simulink model "sim"  (R2022b)
settings: Solver=FixedStepAuto  StartTime=0.0  StopTime=20  FixedStep=0.01  RelTol=1e-3
values from neighbouring files (symbols this model uses):
  A = double(vpa(subs(A, [x, Parameter, u], [xe, Parameter_value, 0]), 10))    [lqr_cartpole.m]
  B = double(vpa(subs(B, [x, Parameter, u], [xe, Parameter_value, 0]), 10))    [lqr_cartpole.m]
  C = double(C)    [lqr_cartpole.m]
  KD = 0.015    [lqr_cartpole.m]
  KP = 0.15    [lqr_cartpole.m]
  L1 = place(A.',C.',poles_ob).'    [lqr_cartpole.m]
undefined symbols (not defined in the file or in its folder): K_LQR
settings Model: Creator=mehti  LastModifiedBy=MMM
settings SolverCC: AlgebraicLoopSolver=TrustRegion
settings DebuggingCC: UnconnectedInputMsg=warning  UnconnectedOutputMsg=warning  UnconnectedLineMsg=warning  SFMachineParentedDataDiag=warning
settings ModelReferenceCC: EnableRefExpFcnMdlSchedulingChecks=on
settings RTWCC: DLArmComputeVersion=19.05

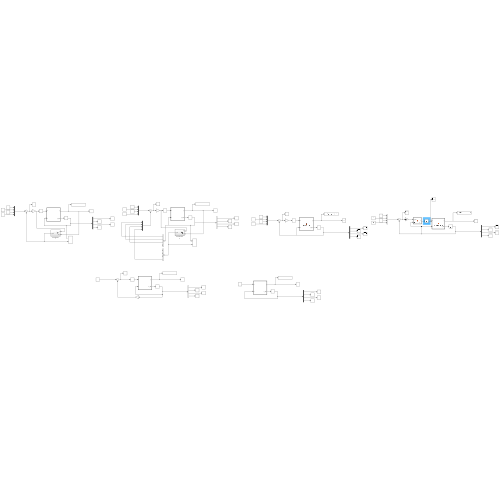
[thumbnail: Simulink's stored preview of the top-level diagram]
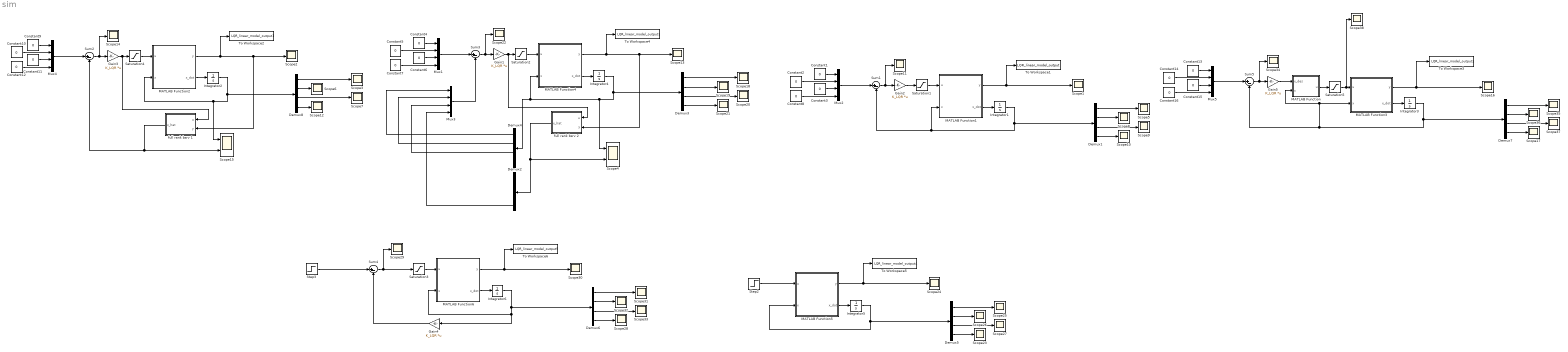
== system sim ==
  Constant{1..16} (16 alike) : Constant  Value=0
  Demux{1..8} (8 alike) : Demux
  Gain{1..5} (5 alike) : Gain  Gain=K_LQR  Multiplication=Matrix(K*u)
  Integrator{1..6} (6 alike) : Integrator  InitialCondition=[0, 0, pi/8 ,0]
  MATLAB Function : MATLAB Function  TreatAsAtomicUnit=on
  MATLAB Function1 : MATLAB Function  TreatAsAtomicUnit=on
  MATLAB Function2 : MATLAB Function  TreatAsAtomicUnit=on
  MATLAB Function3 : MATLAB Function  TreatAsAtomicUnit=on
  MATLAB Function4 : MATLAB Function  TreatAsAtomicUnit=on
  MATLAB Function5 : MATLAB Function  TreatAsAtomicUnit=on
  MATLAB Function6 : MATLAB Function  TreatAsAtomicUnit=on
  Mux{1..5} (5 alike) : Mux
  Saturation{1..4} (4 alike) : Saturate  UpperLimit=10  LowerLimit=-10
  Saturation5 : Saturate  UpperLimit=1000  LowerLimit=-1000
  Scope{1..3,5..14,16..38} (36 alike) : Scope
  Scope15 : Scope  NumInputPorts=2
  Scope4 : Scope  NumInputPorts=2
  Step2 : Step  Time=0.5  After=0  SampleTime=0
  Step3 : Step  Time=0.5  After=0.2  SampleTime=0
  Sum{1..5} (5 alike) : Sum  Inputs=|+-
  To Workspace1 : ToWorkspace  VariableName=LQR_linear_model_output  SaveFormat=Timeseries  SampleTime=-1
  To Workspace2 : ToWorkspace  VariableName=LQR_linear_model_output1  SaveFormat=Timeseries  SampleTime=-1
  To Workspace3 : ToWorkspace  VariableName=LQR_linear_model_output2  SaveFormat=Timeseries  SampleTime=-1
  To Workspace4 : ToWorkspace  VariableName=LQR_linear_model_output3  SaveFormat=Timeseries  SampleTime=-1
  To Workspace5 : ToWorkspace  VariableName=LQR_linear_model_output4  SaveFormat=Timeseries  SampleTime=-1
  To Workspace6 : ToWorkspace  VariableName=LQR_linear_model_output5  SaveFormat=Timeseries  SampleTime=-1
  full rank bsrv 1 : Subsystem
  full rank bsrv 2 : Subsystem
  wires:
  Saturation2/1 -> MATLAB Function4/1(u)
  Constant7/1 -> Mux1/4
  Constant5/1 -> Mux1/2
  Constant6/1 -> Mux1/3
  Constant4/1 -> Mux1/1
  Demux3/1 -> Scope18/1
  Demux3/2 -> Scope19/1
  Demux3/3 -> Scope20/1
  Demux3/4 -> Scope21/1
  Gain1/1 -> full rank bsrv 2/1(u), Saturation2/1
  Integrator4/1 -> Scope4/1, Demux4/1, MATLAB Function4/2(x), Demux3/1
  Sum3/1 -> Gain1/1, Scope22/1
  MATLAB Function4/2(x_dot) -> Integrator4/1
  MATLAB Function4/1(y) -> To Workspace4/1, full rank bsrv 2/2(y), Scope13/1
  Mux1/1 -> Sum3/1
  Step2/1 -> MATLAB Function5/1(u)
  Demux5/1 -> Scope25/1
  Demux5/2 -> Scope26/1
  Demux5/3 -> Scope27/1
  MATLAB Function5/2(x_dot) -> Integrator5/1
  Integrator5/1 -> Demux5/1, MATLAB Function5/2(x)
  Demux5/4 -> Scope23/1
  MATLAB Function5/1(y) -> Scope24/1, To Workspace5/1
  Step3/1 -> Sum4/1
  Gain4/1 -> Sum4/2
  MATLAB Function6/1(y) -> To Workspace6/1, Scope30/1
  Demux6/4 -> Scope28/1
  Integrator6/1 -> MATLAB Function6/2(x), Gain4/1, Demux6/1
  MATLAB Function6/2(x_dot) -> Integrator6/1
  Demux6/3 -> Scope33/1
  Demux6/2 -> Scope32/1
  Saturation3/1 -> MATLAB Function6/1(u)
  Demux6/1 -> Scope31/1
  Sum4/1 -> Scope29/1, Saturation3/1
  full rank bsrv 2/1(x_hat) -> Demux2/1, Scope4/2
  Demux4/1 -> Mux3/1
  Demux4/2 -> Mux3/2
  Demux4/3 -> Mux3/3
  Demux2/4 -> Mux3/4
  Mux3/1 -> Sum3/2
  Constant8/1 -> Mux2/4
  Demux1/2 -> Scope8/1
  Constant2/1 -> Mux2/2
  Saturation1/1 -> MATLAB Function1/1(u)
  Constant3/1 -> Mux2/3
  Constant1/1 -> Mux2/1
  Demux1/3 -> Scope9/1
  Sum1/1 -> Scope11/1, Gain2/1
  Demux1/1 -> Scope5/1
  Integrator1/1 -> Demux1/1, MATLAB Function1/2(x), Sum1/2
  MATLAB Function1/1(y) -> Scope1/1, To Workspace1/1
  Demux1/4 -> Scope10/1
  MATLAB Function1/2(x_dot) -> Integrator1/1
  Gain2/1 -> Saturation1/1
  Mux2/1 -> Sum1/1
  full rank bsrv 1/1(x_hat) -> Sum2/2, Scope15/2
  Mux4/1 -> Sum2/1
  MATLAB Function2/1(y) -> Scope2/1, full rank bsrv 1/2(y), To Workspace2/1
  MATLAB Function2/2(x_dot) -> Integrator2/1
  Sum2/1 -> Scope14/1, Gain3/1
  Integrator2/1 -> Demux8/1, MATLAB Function2/2(x), Scope15/1
  Gain3/1 -> Saturation4/1, full rank bsrv 1/1(u)
  Demux8/4 -> Scope12/1
  Demux8/3 -> Scope7/1
  Demux8/2 -> Scope6/1
  Demux8/1 -> Scope3/1
  Constant9/1 -> Mux4/1
  Constant11/1 -> Mux4/3
  Constant10/1 -> Mux4/2
  Constant12/1 -> Mux4/4
  Saturation4/1 -> MATLAB Function2/1(u)
  Mux5/1 -> Sum5/1
  Gain5/1 -> MATLAB Function/1(x_des)
  MATLAB Function3/2(x_dot) -> Integrator3/1
  Demux7/4 -> Scope17/1
  MATLAB Function3/1(y) -> To Workspace3/1, Scope16/1
  Integrator3/1 -> Sum5/2, MATLAB Function3/2(x), MATLAB Function/2(x), Demux7/1
  Demux7/1 -> Scope35/1
  Sum5/1 -> Gain5/1, Scope34/1
  Demux7/3 -> Scope37/1
  Constant13/1 -> Mux5/1
  Constant15/1 -> Mux5/3
  Saturation5/1 -> Scope38/1, MATLAB Function3/1(u)
  Constant14/1 -> Mux5/2
  Demux7/2 -> Scope36/1
  Constant16/1 -> Mux5/4
  MATLAB Function/1(u) -> Saturation5/1

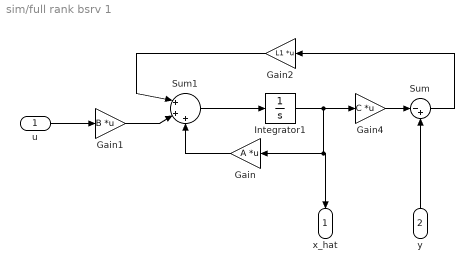
== system sim/full rank bsrv 1 ==
  u : Inport
  y : Inport  Port=2
  Gain : Gain  Gain=A  Multiplication=Matrix(K*u)
  Gain1 : Gain  Gain=B  Multiplication=Matrix(K*u)
  Gain2 : Gain  Gain=L1  Multiplication=Matrix(K*u)
  Gain4 : Gain  Gain=C  Multiplication=Matrix(K*u)
  Integrator1 : Integrator
  Sum : Sum  Inputs=|-+
  Sum1 : Sum  Inputs=|+++
  x_hat : Outport
  wires:
  Gain/1 -> Sum1/3
  Gain2/1 -> Sum1/1
  u/1 -> Gain1/1
  Gain1/1 -> Sum1/2
  Sum/1 -> Gain2/1
  Integrator1/1 -> Gain4/1, x_hat/1, Gain/1
  Gain4/1 -> Sum/1
  Sum1/1 -> Integrator1/1
  y/1 -> Sum/2

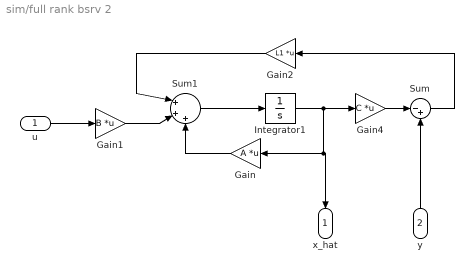
== system sim/full rank bsrv 2 ==
  u : Inport
  y : Inport  Port=2
  Gain : Gain  Gain=A  Multiplication=Matrix(K*u)
  Gain1 : Gain  Gain=B  Multiplication=Matrix(K*u)
  Gain2 : Gain  Gain=L1  Multiplication=Matrix(K*u)
  Gain4 : Gain  Gain=C  Multiplication=Matrix(K*u)
  Integrator1 : Integrator
  Sum : Sum  Inputs=|-+
  Sum1 : Sum  Inputs=|+++
  x_hat : Outport
  wires:
  y/1 -> Sum/2
  Sum1/1 -> Integrator1/1
  Gain4/1 -> Sum/1
  Integrator1/1 -> Gain/1, x_hat/1, Gain4/1
  Sum/1 -> Gain2/1
  Gain1/1 -> Sum1/2
  u/1 -> Gain1/1
  Gain2/1 -> Sum1/1
  Gain/1 -> Sum1/3

== matlab function sim/MATLAB Function1 ==
  data: u input; y output; x input; x_dot output
function [y, x_dot] = nonlinear_model(u, x)

% The state variables
x1 = x(1); x2 = x(2);
x3 = x(3); x4 = x(4);

% Parameters
m_p = 0.2;       % Pendulum mass [kg]
m_w = 0.1;       % mass end of Pendulum [kg]
M = 0.694;           % Cart mass [kg]
l = 0.5;           % Pendulum length [m]
g = 9.8065;  % Gravitational acceleration [m/s^2]

% l is the length of the pole and L is the distance from COM
% m_p is the weight of the pole and m_w is the weirht of the mass

L = (0.5 * m_p + m_w)/(m_p + m_w) * l;
m = m_p + m_w;
I = (1/3 * m_p + m_w) * l^2;
Delta = (I + m*L^2) * (M + m) - (m*L*cos(x3))^2; 


% Nonlinear equations 
x_dot = [x2;
        (1/Delta) * ((I+m*L^2)*(u+m*L*sin(x3)*x4^2)-m^2*L^2*g*sin(x3)*cos(x3));
         x4;
        (1/Delta) * ((m+M)*m*g*L*sin(x3) - m*L*cos(x3)*(m*L*x4^2*sin(x3)+u)); 
          ];

y = [x1;
     x3];

end

== matlab function sim/MATLAB Function2 ==
  data: u input; y output; x input; x_dot output
function [y, x_dot] = nonlinear_model(u, x)

% The state variables
x1 = x(1); x2 = x(2);
x3 = x(3); x4 = x(4);

% Parameters
m_p = 0.2;       % Pendulum mass [kg]
m_w = 0.1;       % mass end of Pendulum [kg]
M = 0.694;           % Cart mass [kg]
l = 0.5;           % Pendulum length [m]
g = 9.8065;  % Gravitational acceleration [m/s^2]

% l is the length of the pole and L is the distance from COM
% m_p is the weight of the pole and m_w is the weirht of the mass

L = (0.5 * m_p + m_w)/(m_p + m_w) * l;
m = m_p + m_w;
I = (1/3 * m_p + m_w) * l^2;
Delta = (I + m*L^2) * (M + m) - (m*L*cos(x3))^2; 


% Nonlinear equations 
x_dot = [x2;
        (1/Delta) * ((I+m*L^2)*(u+m*L*sin(x3)*x4^2)-m^2*L^2*g*sin(x3)*cos(x3));
         x4;
        (1/Delta) * ((m+M)*m*g*L*sin(x3) - m*L*cos(x3)*(m*L*x4^2*sin(x3)+u)); 
          ];

y = [x1;
     x3];

end

== matlab function sim/MATLAB Function3 ==
  data: u input; y output; x input; x_dot output
function [y, x_dot] = nonlinear_model(u, x)

% The state variables
x1 = x(1); x2 = x(2);
x3 = x(3); x4 = x(4);

% Parameters
m_p = 0.2;       % Pendulum mass [kg]
m_w = 0.1;       % mass end of Pendulum [kg]
M = 0.694;           % Cart mass [kg]
l = 0.5;           % Pendulum length [m]
g = 9.8065;  % Gravitational acceleration [m/s^2]

% l is the length of the pole and L is the distance from COM
% m_p is the weight of the pole and m_w is the weirht of the mass

L = (0.5 * m_p + m_w)/(m_p + m_w) * l;
m = m_p + m_w;
I = (1/3 * m_p + m_w) * l^2;
Delta = (I + m*L^2) * (M + m) - (m*L*cos(x3))^2; 


% Nonlinear equations 
x_dot = [x2;
        (1/Delta) * ((I+m*L^2)*(u+m*L*sin(x3)*x4^2)-m^2*L^2*g*sin(x3)*cos(x3));
         x4;
        (1/Delta) * ((m+M)*m*g*L*sin(x3) - m*L*cos(x3)*(m*L*x4^2*sin(x3)+u)); 
          ];

y = [x1;
     x3];

end

== matlab function sim/MATLAB Function4 ==
  data: u input; y output; x input; x_dot output
function [y, x_dot] = nonlinear_model(u, x)

% The state variables
x1 = x(1); x2 = x(2);
x3 = x(3); x4 = x(4);

% Parameters
m_p = 0.2;       % Pendulum mass [kg]
m_w = 0.1;       % mass end of Pendulum [kg]
M = 0.694;           % Cart mass [kg]
l = 0.5;           % Pendulum length [m]
g = 9.8065;  % Gravitational acceleration [m/s^2]

% l is the length of the pole and L is the distance from COM
% m_p is the weight of the pole and m_w is the weirht of the mass

L = (0.5 * m_p + m_w)/(m_p + m_w) * l;
m = m_p + m_w;
I = (1/3 * m_p + m_w) * l^2;
Delta = (I + m*L^2) * (M + m) - (m*L*cos(x3))^2; 


% Nonlinear equations 
x_dot = [x2;
        (1/Delta) * ((I+m*L^2)*(u+m*L*sin(x3)*x4^2)-m^2*L^2*g*sin(x3)*cos(x3));
         x4;
        (1/Delta) * ((m+M)*m*g*L*sin(x3) - m*L*cos(x3)*(m*L*x4^2*sin(x3)+u)); 
          ];

y = [x1;
     x3];

end

== matlab function sim/MATLAB Function5 ==
  data: u input; y output; x input; x_dot output
function [y, x_dot] = nonlinear_model(u, x)

% The state variables
x1 = x(1); x2 = x(2);
x3 = x(3); x4 = x(4);

% Parameters
m_p = 0.2;       % Pendulum mass [kg]
m_w = 0.1;       % mass end of Pendulum [kg]
M = 0.694;           % Cart mass [kg]
l = 0.5;           % Pendulum length [m]
g = 9.8065;  % Gravitational acceleration [m/s^2]

% l is the length of the pole and L is the distance from COM
% m_p is the weight of the pole and m_w is the weirht of the mass

L = (0.5 * m_p + m_w)/(m_p + m_w) * l;
m = m_p + m_w;
I = (1/3 * m_p + m_w) * l^2;
Delta = (I + m*L^2) * (M + m) - (m*L*cos(x3))^2; 


% Nonlinear equations 
x_dot = [x2;
        (1/Delta) * ((I+m*L^2)*(u+m*L*sin(x3)*x4^2)-m^2*L^2*g*sin(x3)*cos(x3));
         x4;
        (1/Delta) * ((m+M)*m*g*L*sin(x3) - m*L*cos(x3)*(m*L*x4^2*sin(x3)+u)); 
          ];

y = [x1;
     x3];

end

== matlab function sim/MATLAB Function6 ==
  data: u input; y output; x input; x_dot output
function [y, x_dot] = nonlinear_model(u, x)

% The state variables
x1 = x(1); x2 = x(2);
x3 = x(3); x4 = x(4);

% Parameters
m_p = 0.2;       % Pendulum mass [kg]
m_w = 0.1;       % mass end of Pendulum [kg]
M = 0.694;           % Cart mass [kg]
l = 0.5;           % Pendulum length [m]
g = 9.8065;  % Gravitational acceleration [m/s^2]

% l is the length of the pole and L is the distance from COM
% m_p is the weight of the pole and m_w is the weirht of the mass

L = (0.5 * m_p + m_w)/(m_p + m_w) * l;
m = m_p + m_w;
I = (1/3 * m_p + m_w) * l^2;
Delta = (I + m*L^2) * (M + m) - (m*L*cos(x3))^2; 


% Nonlinear equations 
x_dot = [x2;
        (1/Delta) * ((I+m*L^2)*(u+m*L*sin(x3)*x4^2)-m^2*L^2*g*sin(x3)*cos(x3));
         x4;
        (1/Delta) * ((m+M)*m*g*L*sin(x3) - m*L*cos(x3)*(m*L*x4^2*sin(x3)+u)); 
          ];

y = [x1;
     x3];

end

== matlab function sim/MATLAB Function ==
  data: x_des input; x input; u output; KP parameter; KD parameter
function u = PD_control(x_des, x, KP, KD)
    % x(1): current position
    % x(2): current velocity
    % KP: proportional gain
    % KD: derivative gain
    % x_des: desired position from LQR
    u = KP * (x_des - x(1)) - KD * x(2);
end
